simulink model "arduinomega2560_drive_openloop"  (Simulink 10.0)
settings: Solver=ode3  StartTime=0.0  StopTime=inf  RelTol=1e-3
InitFcn:
  | lego_drive_openloop_InitData.mdl = get_param(bdroot,'Name');
  | lego_drive_openloop_InitData.cs = getActiveConfigSet(lego_drive_openloop_InitData.mdl);
libraries: arduinolib x8, simulink x1
PreSaveFcn:
  | set_param(gcs, 'location', [45 95 785 420])
CloseFcn:
  | clear lego_drive_openloop_InitData
settings Model: Creator=The MathWorks Inc.  LastModifiedBy=bhisma  ExtModeTrigDuration=2
settings DataIOCC: LimitDataPoints=on  SignalLoggingSaveFormat=ModelDataLogs
settings OptimizationCC: ExpressionDepthLimit=2147483647  LifeSpan=1  EfficientTunableParamExpr=on
settings DebuggingCC: InheritedTsInSrcMsg=none  ParameterPrecisionLossMsg=none  FcnCallInpInsideContextMsg=warning  StateNameClashWarn=warning
settings HardwareCC: ProdBitPerInt=16  ProdBitPerPointer=16  ProdBitPerSizeT=16  ProdBitPerPtrDiffT=16  ProdIntDivRoundTo=Zero  ProdEndianess=LittleEndian  ProdWordSize=8  ProdHWDeviceType=Atmel->AVR
settings SFSimCC: MATLABDynamicMemAlloc=off
settings RTWCC: Description=Real-Time Toolbox  SystemTargetFile=realtime.tlc  GenerateMakefile=off  TemplateMakefile=realtime.tmf  RTWVerbose=off
settings CodeAppCC: CustomSymbolStrType=$N$R$M  InternalIdentifier=Classic
settings STFCustomTargetCC: TargetLibSuffix=.a  GenerateSampleERTMain=on  ERTCustomFileBanners=on  SupportNonInlinedSFcns=off  RemoveResetFunc=on  SupportVariableSizeSignals=on  MATLABClassNameForMDSCustomization=Simulink.SoftwareTarget.ERTCustomization  GRTInterface=off  SystemTargetFile=realtime.tlc
settings ERTTargetCC: MultiwordLength=2048  GenerateSampleERTMain=on  ParMdlRefBuildCompliant=off  CompOptLevelCompliant=off  ConcurrentExecutionCompliant=off  CombineOutputUpdateFcns=off  SupportContinuousTime=on  SupportVariableSizeSignals=on  ModelStepFunctionPrototypeControlCompliant=off  CPPClassGenCompliant=off  UseToolchainInfoCompliant=off  ExtModeTransport=3  ExtModeMexFile=ext_serial_win32_comm  ExtModeMexArgs=0 1 115200  ERTSrcFileBannerTemplate=realtime_code_template.cgt  ERTHdrFileBannerTemplate=realtime_code_template.cgt  ERTDataSrcFileTemplate=realtime_code_template.cgt  ERTDataHdrFileTemplate=realtime_code_template.cgt  ERTCustomFileTemplate=realtime_file_process.tlc  ConvertIfToSwitch=off  SuppressUnreachableDefaultCases=off
settings ConfigComp: CovExternalEMLEnable=off
settings SettingsController: Description=Run on Hardware Dialog  TargetExtensionPlatform=Arduino Mega 2560
settings MATStruct: Set_host_COM_port=[0.0]  COM_port_number=1  COM_port_baud_rate=115200  Enable_overrun_detection=[0.0]  Digital_output_to_set_on_overrun=13  Analog_input_reference_voltage=[0.0]  Serial1_baud_rate=9600  Serial2_baud_rate=9600  Serial3_baud_rate=9600  Serial0_baud_rate=115200

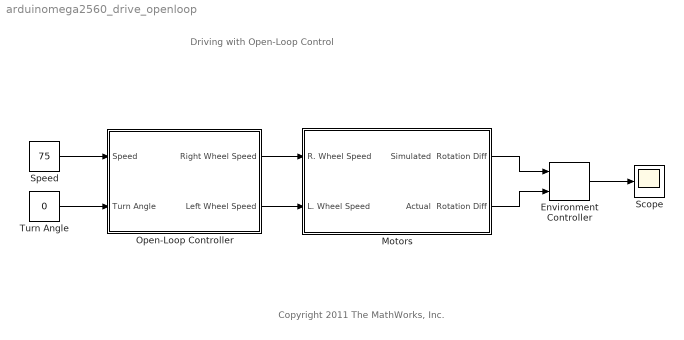
== system arduinomega2560_drive_openloop ==
  note: Copyright 2011 The MathWorks, Inc.
  note: Driving with Open-Loop Control
  Environment Controller : simulink/Signal Routing/Environment Controller
      settings: SourceProductName=Simulink  SourceProductBaseCode=SL
  Motors : Subsystem  VariantControl=DoSim
  Open-Loop Controller : Subsystem
  Scope : Scope
  Speed : Constant  Value=75  OutMin=0  OutMax=100  OutDataTypeStr=single  SampleTime=0.001
  Turn Angle : Constant  Value=0  OutMin=-50  OutMax=50  OutDataTypeStr=single  SampleTime=0.001
  wires:
  Speed/1 -> Open-Loop Controller/1(Speed)
  Turn Angle/1 -> Open-Loop Controller/2(Turn Angle)
  Open-Loop Controller/1(Right Wheel Speed) -> Motors/1(R. Wheel Speed)
  Open-Loop Controller/2(Left Wheel Speed) -> Motors/2(L. Wheel Speed)
  Environment Controller/1 -> Scope/1
  Motors/1(Simulated  Rotation Diff) -> Environment Controller/1
  Motors/2(Actual  Rotation Diff) -> Environment Controller/2

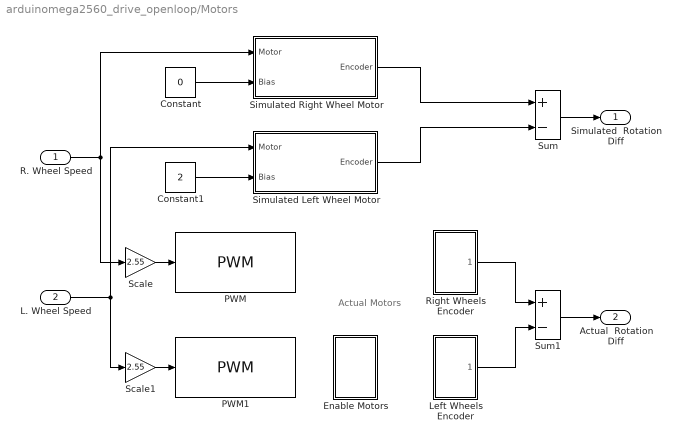
== system arduinomega2560_drive_openloop/Motors ==
  note: Actual
      | Motors
  R. Wheel Speed : Inport
  L. Wheel Speed : Inport  Port=2
  Constant : Constant  Value=0  OutDataTypeStr=single
  Constant1 : Constant  Value=2  OutDataTypeStr=single
  Enable Motors : Subsystem
  Left Wheels Encoder : Subsystem
  PWM : arduinolib/PWM  pinNumber=10
  PWM1 : arduinolib/PWM  pinNumber=11
  Right Wheels Encoder : Subsystem
  Scale : Gain  Gain=2.55
  Scale1 : Gain  Gain=2.55
  Simulated Left Wheel Motor : Subsystem
  Simulated Right Wheel Motor : Subsystem
  Sum : Sum  Inputs=+-  OutDataTypeStr=Inherit: Same as first input
  Sum1 : Sum  Inputs=+-  OutDataTypeStr=Inherit: Same as first input
  Simulated  Rotation Diff : Outport
  Actual  Rotation Diff : Outport  Port=2
  wires:
  Sum1/1 -> Actual  Rotation Diff/1
  Sum/1 -> Simulated  Rotation Diff/1
  Simulated Left Wheel Motor/1(Encoder) -> Sum/2
  Simulated Right Wheel Motor/1(Encoder) -> Sum/1
  R. Wheel Speed/1 -> Simulated Right Wheel Motor/1(Motor), Scale/1
  L. Wheel Speed/1 -> Simulated Left Wheel Motor/1(Motor), Scale1/1
  Constant/1 -> Simulated Right Wheel Motor/2(Bias)
  Constant1/1 -> Simulated Left Wheel Motor/2(Bias)
  Left Wheels Encoder/1(Encoder) -> Sum1/2
  Right Wheels Encoder/1(Encoder) -> Sum1/1
  Scale/1 -> PWM/1
  Scale1/1 -> PWM1/1

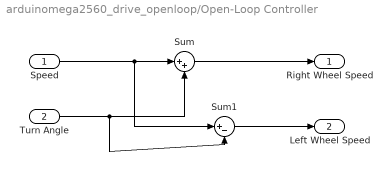
== system arduinomega2560_drive_openloop/Open-Loop Controller ==
  Speed : Inport
  Turn Angle : Inport  Port=2
  Sum : Sum  Inputs=|++  OutDataTypeStr=Inherit: Same as first input
  Sum1 : Sum  Inputs=|+-  OutDataTypeStr=Inherit: Same as first input
  Right Wheel Speed : Outport
  Left Wheel Speed : Outport  Port=2
  wires:
  Sum1/1 -> Left Wheel Speed/1
  Sum/1 -> Right Wheel Speed/1
  Turn Angle/1 -> Sum1/2, Sum/2
  Speed/1 -> Sum1/1, Sum/1

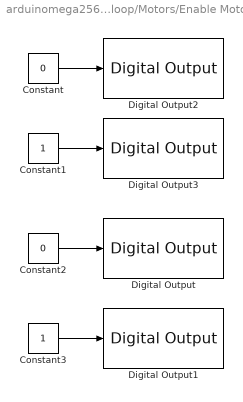
== system arduinomega2560_drive_openloop/Motors/Enable Motors ==
  Constant : Constant  Value=0  OutDataTypeStr=boolean
  Constant1 : Constant  OutDataTypeStr=boolean
  Constant2 : Constant  Value=0  OutDataTypeStr=boolean
  Constant3 : Constant  OutDataTypeStr=boolean
  Digital Output : arduinolib/Digital Output  pinNumber=2
  Digital Output1 : arduinolib/Digital Output  pinNumber=3
  Digital Output2 : arduinolib/Digital Output  pinNumber=4
  Digital Output3 : arduinolib/Digital Output  pinNumber=5
  wires:
  Constant1/1 -> Digital Output3/1
  Constant/1 -> Digital Output2/1
  Constant2/1 -> Digital Output/1
  Constant3/1 -> Digital Output1/1

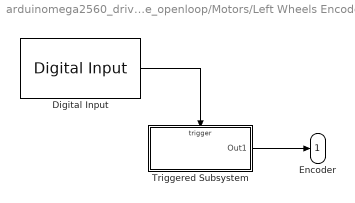
== system arduinomega2560_drive_openloop/Motors/Left Wheels Encoder ==
  Digital Input : arduinolib/Digital Input  pinNumber=9  sampleTime=0.001
      settings: SourceProductName=Simulink Support Package for Arduino Hardware
  Triggered Subsystem : Subsystem  TreatAsAtomicUnit=on
  Encoder : Outport
  wires:
  Digital Input/1 -> Triggered Subsystem/Trigger
  Triggered Subsystem/1(Out1) -> Encoder/1

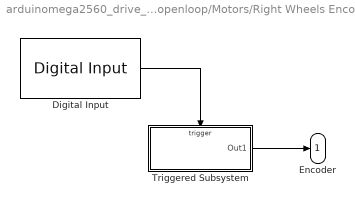
== system arduinomega2560_drive_openloop/Motors/Right Wheels Encoder ==
  Digital Input : arduinolib/Digital Input  pinNumber=8  sampleTime=0.001
      settings: SourceProductName=Simulink Support Package for Arduino Hardware
  Triggered Subsystem : Subsystem  TreatAsAtomicUnit=on
  Encoder : Outport
  wires:
  Triggered Subsystem/1(Out1) -> Encoder/1
  Digital Input/1 -> Triggered Subsystem/Trigger

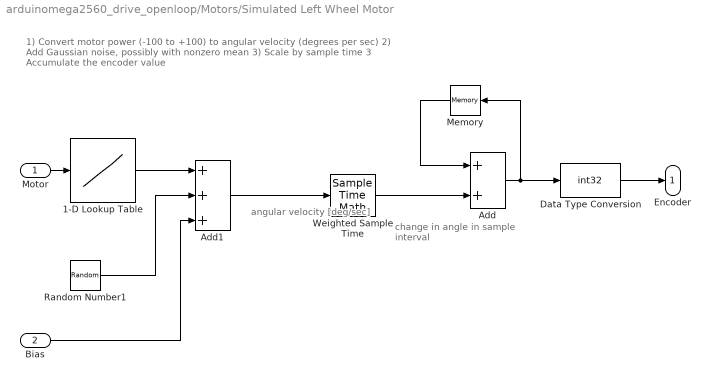
== system arduinomega2560_drive_openloop/Motors/Simulated Left Wheel Motor ==
  note: change in angle
      | in sample interval
  note: angular velocity
      | [deg/sec]
  note: 1) Convert motor power (-100 to +100) to angular velocity (degrees per sec)
      | 2) Add Gaussian noise, possibly with nonzero mean
      | 3) Scale by sample time
      | 3 Accumulate the encoder value
  Motor : Inport
  Bias : Inport  Port=2
  1-D Lookup Table : Lookup_n-D  NumberOfTableDimensions=1  BreakpointsForDimension1=[-100 0 100]  Table=[-360 0 360]  ExtrapMethod=Clip  UseLastTableValue=on  RndMeth=Simplest  InputSameDT=on
  Add : Sum  OutDataTypeStr=Inherit: Same as first input
  Add1 : Sum  Inputs=+++  OutDataTypeStr=single
  Data Type Conversion : DataTypeConversion  OutDataTypeStr=int32
  Memory : Memory  InheritSampleTime=on  LinearizeAsDelay=on
  Random Number1 : RandomNumber  Variance=5  Seed=randi(1000)
  Weighted Sample Time : SampleTimeMath  TsampMathOp=*
  Encoder : Outport
  wires:
  Data Type Conversion/1 -> Encoder/1
  Bias/1 -> Add1/3
  Weighted Sample Time/1 -> Add/2
  Add/1 -> Data Type Conversion/1, Memory/1
  Memory/1 -> Add/1
  Add1/1 -> Weighted Sample Time/1
  Motor/1 -> 1-D Lookup Table/1
  Random Number1/1 -> Add1/2
  1-D Lookup Table/1 -> Add1/1

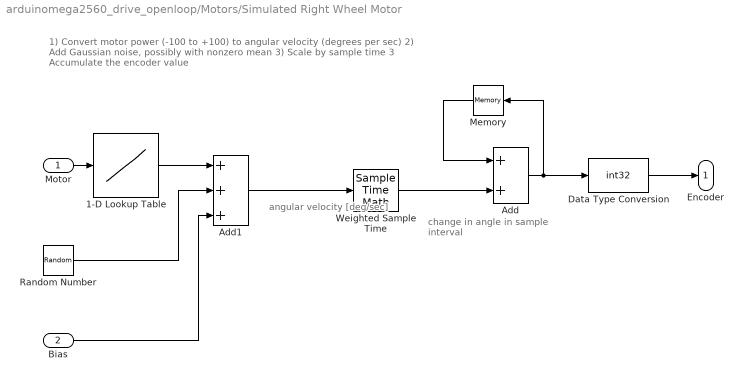
== system arduinomega2560_drive_openloop/Motors/Simulated Right Wheel Motor ==
  note: 1) Convert motor power (-100 to +100) to angular velocity (degrees per sec)
      | 2) Add Gaussian noise, possibly with nonzero mean
      | 3) Scale by sample time
      | 3 Accumulate the encoder value
  note: angular velocity
      |  [deg/sec]
  note: change in angle
      | in sample interval
  Motor : Inport
  Bias : Inport  Port=2
  1-D Lookup Table : Lookup_n-D  NumberOfTableDimensions=1  BreakpointsForDimension1=[-100 0 100]  Table=[-360 0 360]  ExtrapMethod=Clip  UseLastTableValue=on  RndMeth=Simplest  InputSameDT=on
  Add : Sum  AccumDataTypeStr=single  OutDataTypeStr=single
  Add1 : Sum  Inputs=+++  OutDataTypeStr=single
  Data Type Conversion : DataTypeConversion  OutDataTypeStr=int32
  Memory : Memory  InheritSampleTime=on  LinearizeAsDelay=on
  Random Number : RandomNumber  Variance=5  Seed=randi(1000)
  Weighted Sample Time : SampleTimeMath  TsampMathOp=*
  Encoder : Outport
  wires:
  Data Type Conversion/1 -> Encoder/1
  1-D Lookup Table/1 -> Add1/1
  Random Number/1 -> Add1/2
  Motor/1 -> 1-D Lookup Table/1
  Memory/1 -> Add/1
  Add/1 -> Data Type Conversion/1, Memory/1
  Weighted Sample Time/1 -> Add/2
  Bias/1 -> Add1/3
  Add1/1 -> Weighted Sample Time/1

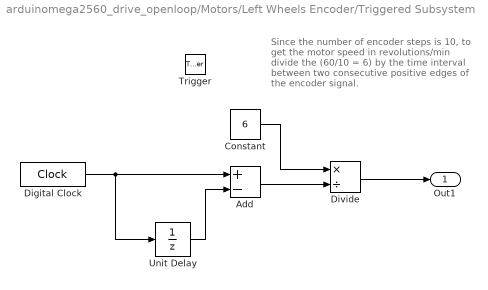
== system arduinomega2560_drive_openloop/Motors/Left Wheels Encoder/Triggered Subsystem ==
  note: Since the number of encoder steps is 10,
      | to get the motor speed in revolutions/min
      | divide the (60/10 = 6) by the time interval
      | between two consecutive positive edges
      | of the encoder signal.
  Trigger : TriggerPort  VariantControl=(inherit)
  Add : Sum  Inputs=+-
  Constant : Constant  Value=6
  Digital Clock : DigitalClock  SampleTime=-1
  Divide : Product  Inputs=*/  OutDataTypeStr=int32
  Unit Delay : UnitDelay  SampleTime=-1  HasFrameUpgradeWarning=on
  Out1 : Outport
  wires:
  Constant/1 -> Divide/1
  Divide/1 -> Out1/1
  Add/1 -> Divide/2
  Unit Delay/1 -> Add/2
  Digital Clock/1 -> Unit Delay/1, Add/1

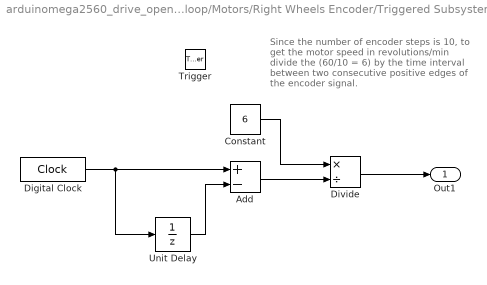
== system arduinomega2560_drive_openloop/Motors/Right Wheels Encoder/Triggered Subsystem ==
  note: Since the number of encoder steps is 10,
      | to get the motor speed in revolutions/min
      | divide the (60/10 = 6) by the time interval
      | between two consecutive positive edges
      | of the encoder signal.
  Trigger : TriggerPort  VariantControl=(inherit)
  Add : Sum  Inputs=+-
  Constant : Constant  Value=6
  Digital Clock : DigitalClock  SampleTime=-1
  Divide : Product  Inputs=*/  OutDataTypeStr=int32
  Unit Delay : UnitDelay  SampleTime=-1  HasFrameUpgradeWarning=on
  Out1 : Outport
  wires:
  Digital Clock/1 -> Add/1, Unit Delay/1
  Unit Delay/1 -> Add/2
  Add/1 -> Divide/2
  Divide/1 -> Out1/1
  Constant/1 -> Divide/1
